simulink model "GMRforHapticsGuidance"  (R2012b)
settings: Solver=ode45  StartTime=0.0  StopTime=3  RelTol=1e-3
values from neighbouring files (symbols this model uses):
  sigmaGMR = [0.000145098551996 2.44735832162e-06 2.27908651022e-05 6.0139473564e-05 -2.08735404133e-05 -5.10583896034e-05 2.73525383282e-05 2.14077979945e-05 2.94117888322e-06 2.44735832162e-06 0.000208854387423 -0.000180360868853 ... (1134 elements, 9x9x14)]    [GMMData.mat]    (also in ModelTraining.m = reshape( covMatrices, [ numVar numVar 1 * numGauss ] ); ModelTraining2gestures.m = sigma; ModelTraining2gesturesZoom.m = sigma; ModelTraining2gesturesv1.m = sigma)
undefined symbols (not defined in the file or in its folder): B1, sigbuilder_block
settings Model: Creator=cperez  LastModifiedBy=andre
settings DataIOCC: SignalLoggingSaveFormat=ModelDataLogs
settings OptimizationCC: ExpressionDepthLimit=128
settings DebuggingCC: MultiTaskDSMMsg=warning  MultiTaskCondExecSysMsg=none  StateNameClashWarn=none  StrictBusMsg=None
settings RTWCC: IncludeERTFirstTime=on
settings CodeAppCC: CustomSymbolStrType=$N$R$M_T  InternalIdentifier=Shortened

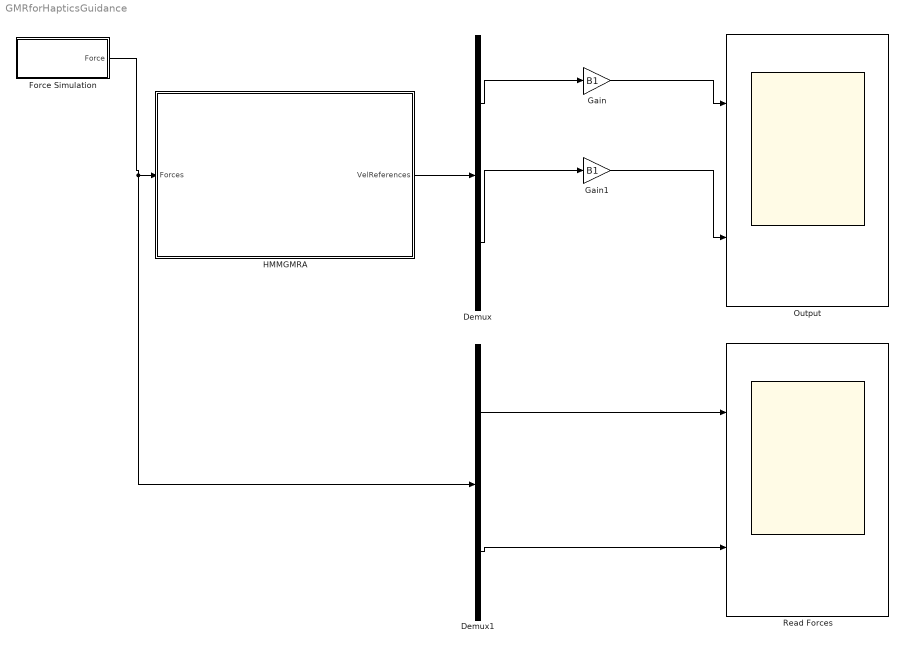
== system GMRforHapticsGuidance ==
  Demux : Demux  Outputs=2
  Demux1 : Demux  Outputs=2
  Force Simulation : Subsystem
  Gain : Gain  Gain=B1
  Gain1 : Gain  Gain=B1
  HMMGMRA : Subsystem
  Output : Scope  NumInputPorts=2
      settings: YMin=-5~-5  YMax=5~5
  Read Forces : Scope  NumInputPorts=2
      settings: YMin=-5~-5  YMax=5~5
  wires:
  HMMGMRA/1(VelReferences) -> Demux/1
  Demux/1 -> Gain/1
  Demux/2 -> Gain1/1
  Gain/1 -> Output/1
  Gain1/1 -> Output/2
  Demux1/1 -> Read Forces/1
  Demux1/2 -> Read Forces/2
  Force Simulation/1(Force) -> Demux1/1, HMMGMRA/1(Forces)

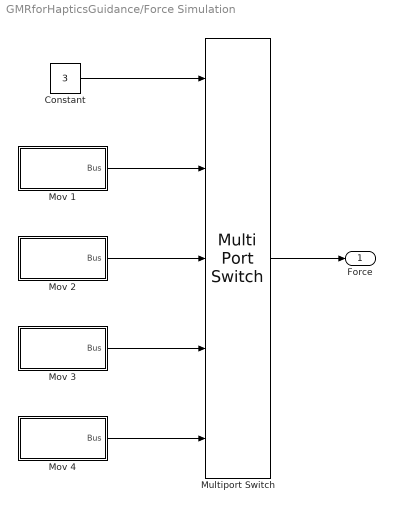
== system GMRforHapticsGuidance/Force Simulation ==
  Constant : Constant  Value=3
  Mov 1 : Subsystem  Tag=STV Subsys  LoadFcn=sigbuilder_block('load');  StartFcn=sigbuilder_block('start');  StopFcn=sigbuilder_block('stop');  ClipboardFcn=sigbuilder_block('clipboard');  mask(Sigbuilder block){}
      mask help: Simulink:masks:SigbuilderBlock_MD
      mask init:
      | if ~strcmp(get_param(bdroot(gcbh),'SimulationStatus'),'stopped') tuvar = sigbuilder_block('maskInit'); end
      settings: CopyFcn=sigbuilder_block('copy');  DeleteFcn=sigbuilder_block('delete');  ModelCloseFcn=sigbuilder_block('modelClose');  PreSaveFcn=sigbuilder_block('preSave');  PauseFcn=sigbuilder_block('pause');  ContinueFcn=sigbuilder_block('continue');  NameChangeFcn=sigbuilder_block('namechange');  OpenFcn=sigbuilder_block('open',[6 28.5 1428 718.5 ]);  CloseFcn=sigbuilder_block('close');
      mask Display: plot(0, 0, 100, 100,[2, 2, 32, 32, 2], [68, 8, 8, 68, 68],[32, 2], [38, 38], [32, 19, 2],[53, 60, 44], [32, 17, 17, 2],[16, 16, 31, 31]);txt = getActiveGroup(gcbh);text(2, 100, txt,'verticalAlignment', 'top');
  Mov 2 : Subsystem  Tag=STV Subsys  LoadFcn=sigbuilder_block('load');  StartFcn=sigbuilder_block('start');  StopFcn=sigbuilder_block('stop');  ClipboardFcn=sigbuilder_block('clipboard');  mask(Sigbuilder block){}
      mask help: Simulink:masks:SigbuilderBlock_MD
      mask init:
      | if ~strcmp(get_param(bdroot(gcbh),'SimulationStatus'),'stopped') tuvar = sigbuilder_block('maskInit'); end
      settings: CopyFcn=sigbuilder_block('copy');  DeleteFcn=sigbuilder_block('delete');  ModelCloseFcn=sigbuilder_block('modelClose');  PreSaveFcn=sigbuilder_block('preSave');  PauseFcn=sigbuilder_block('pause');  ContinueFcn=sigbuilder_block('continue');  NameChangeFcn=sigbuilder_block('namechange');  OpenFcn=sigbuilder_block('open',[6 28.5 1428 718.5 ]);  CloseFcn=sigbuilder_block('close');
      mask Display: plot(0, 0, 100, 100,[2, 2, 32, 32, 2], [68, 8, 8, 68, 68],[32, 2], [38, 38], [32, 19, 2],[53, 60, 44], [32, 17, 17, 2],[16, 16, 31, 31]);txt = getActiveGroup(gcbh);text(2, 100, txt,'verticalAlignment', 'top');
  Mov 3 : Subsystem  Tag=STV Subsys  LoadFcn=sigbuilder_block('load');  StartFcn=sigbuilder_block('start');  StopFcn=sigbuilder_block('stop');  ClipboardFcn=sigbuilder_block('clipboard');  mask(Sigbuilder block){}
      mask help: Simulink:masks:SigbuilderBlock_MD
      mask init:
      | if ~strcmp(get_param(bdroot(gcbh),'SimulationStatus'),'stopped') tuvar = sigbuilder_block('maskInit'); end
      settings: CopyFcn=sigbuilder_block('copy');  DeleteFcn=sigbuilder_block('delete');  ModelCloseFcn=sigbuilder_block('modelClose');  PreSaveFcn=sigbuilder_block('preSave');  PauseFcn=sigbuilder_block('pause');  ContinueFcn=sigbuilder_block('continue');  NameChangeFcn=sigbuilder_block('namechange');  OpenFcn=sigbuilder_block('open',[6 28.5 1428 718.5 ]);  CloseFcn=sigbuilder_block('close');
      mask Display: plot(0, 0, 100, 100,[2, 2, 32, 32, 2], [68, 8, 8, 68, 68],[32, 2], [38, 38], [32, 19, 2],[53, 60, 44], [32, 17, 17, 2],[16, 16, 31, 31]);txt = getActiveGroup(gcbh);text(2, 100, txt,'verticalAlignment', 'top');
  Mov 4 : Subsystem  Tag=STV Subsys  LoadFcn=sigbuilder_block('load');  StartFcn=sigbuilder_block('start');  StopFcn=sigbuilder_block('stop');  ClipboardFcn=sigbuilder_block('clipboard');  mask(Sigbuilder block){}
      mask help: Simulink:masks:SigbuilderBlock_MD
      mask init:
      | if ~strcmp(get_param(bdroot(gcbh),'SimulationStatus'),'stopped') tuvar = sigbuilder_block('maskInit'); end
      settings: CopyFcn=sigbuilder_block('copy');  DeleteFcn=sigbuilder_block('delete');  ModelCloseFcn=sigbuilder_block('modelClose');  PreSaveFcn=sigbuilder_block('preSave');  PauseFcn=sigbuilder_block('pause');  ContinueFcn=sigbuilder_block('continue');  NameChangeFcn=sigbuilder_block('namechange');  OpenFcn=sigbuilder_block('open',[6 28.5 1428 718.5 ]);  CloseFcn=sigbuilder_block('close');
      mask Display: plot(0, 0, 100, 100,[2, 2, 32, 32, 2], [68, 8, 8, 68, 68],[32, 2], [38, 38], [32, 19, 2],[53, 60, 44], [32, 17, 17, 2],[16, 16, 31, 31]);txt = getActiveGroup(gcbh);text(2, 100, txt,'verticalAlignment', 'top');
  Multiport Switch : MultiPortSwitch  Inputs=4
  Force : Outport
  wires:
  Multiport Switch/1 -> Force/1
  Constant/1 -> Multiport Switch/1
  Mov 1/1(Bus) -> Multiport Switch/2
  Mov 2/1(Bus) -> Multiport Switch/3
  Mov 3/1(Bus) -> Multiport Switch/4
  Mov 4/1(Bus) -> Multiport Switch/5

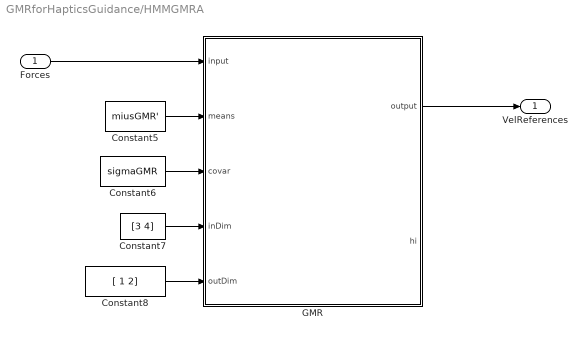
== system GMRforHapticsGuidance/HMMGMRA ==
  Forces : Inport
  Constant5 : Constant  Value=miusGMR'
  Constant6 : Constant  Value=sigmaGMR
  Constant7 : Constant  Value=[3 4]
  Constant8 : Constant  Value=[ 1 2]
  GMR : MATLAB Function  TreatAsAtomicUnit=on
  VelReferences : Outport
  wires:
  GMR/1(output) -> VelReferences/1
  Forces/1 -> GMR/1(input)
  Constant5/1 -> GMR/2(means)
  Constant6/1 -> GMR/3(covar)
  Constant7/1 -> GMR/4(inDim)
  Constant8/1 -> GMR/5(outDim)

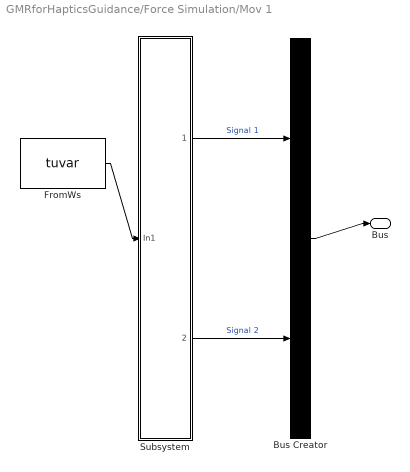
== system GMRforHapticsGuidance/Force Simulation/Mov 1 ==
  Bus Creator : BusCreator  Tag=Bus Creator  Inputs=2
  FromWs : FromWorkspace  Tag=STV FromWs  VariableName=tuvar  SampleTime=0
      SigBuilderData=|
      | common.afterFinalStr = 'Extrapolate'
      | common.sampleTime = 0
      | dataSet.timeRange = [0 3]
      | dataSet.name = 'Group 1'
      | sbobj.Groups.Name = 'Group 1'
      | sbobj.Groups.Signals(1).Name = 'Signal 1'
      | sbobj.Groups.Signals(1).XData = [0 3]
      | sbobj.Groups.Signals(1).YData = [2 0]
      | sbobj.Groups.Signals(2).Name = 'Signal 2'
      | sbobj.Groups.Signals(2).XData = [0 3]
      | sbobj.Groups.Signals(2).YData = [0 0]
      | sbobj.Groups.TimeRange = [0 3]
  Subsystem : Subsystem
  Bus : Outport
  wires:
  FromWs/1 -> Subsystem/1(In1)
  Subsystem/1(Signal 1) -> Bus Creator/1  "Signal 1"
  Subsystem/2(Signal 2) -> Bus Creator/2  "Signal 2"
  Bus Creator/1 -> Bus/1

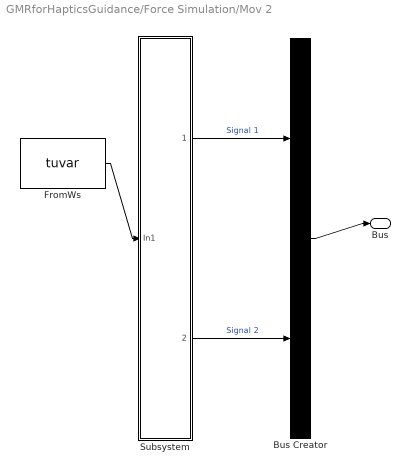
== system GMRforHapticsGuidance/Force Simulation/Mov 2 ==
  Bus Creator : BusCreator  Tag=Bus Creator  Inputs=2
  FromWs : FromWorkspace  Tag=STV FromWs  VariableName=tuvar  SampleTime=0
      SigBuilderData=|
      | common.afterFinalStr = 'Extrapolate'
      | common.sampleTime = 0
      | dataSet.timeRange = [0 3]
      | dataSet.name = 'Group 1'
      | sbobj.Groups.Name = 'Group 1'
      | sbobj.Groups.Signals(1).Name = 'Signal 1'
      | sbobj.Groups.Signals(1).XData = [0 3]
      | sbobj.Groups.Signals(1).YData = [-2 0]
      | sbobj.Groups.Signals(2).Name = 'Signal 2'
      | sbobj.Groups.Signals(2).XData = [0 3]
      | sbobj.Groups.Signals(2).YData = [0 0]
      | sbobj.Groups.TimeRange = [0 3]
  Subsystem : Subsystem
  Bus : Outport
  wires:
  FromWs/1 -> Subsystem/1(In1)
  Subsystem/1(Signal 1) -> Bus Creator/1  "Signal 1"
  Subsystem/2(Signal 2) -> Bus Creator/2  "Signal 2"
  Bus Creator/1 -> Bus/1

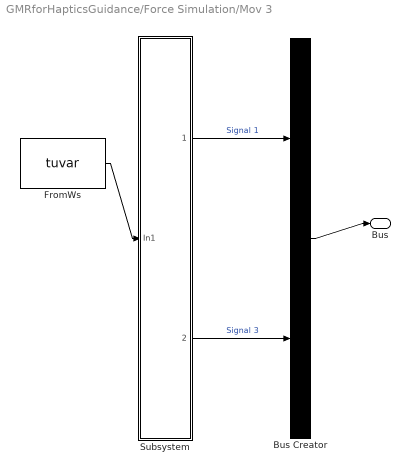
== system GMRforHapticsGuidance/Force Simulation/Mov 3 ==
  Bus Creator : BusCreator  Tag=Bus Creator  Inputs=2
  FromWs : FromWorkspace  Tag=STV FromWs  VariableName=tuvar  SampleTime=0
      SigBuilderData=|
      | common.afterFinalStr = 'Extrapolate'
      | common.sampleTime = 0
      | dataSet.timeRange = [0 3]
      | dataSet.name = 'Group 1'
      | sbobj.Groups.Name = 'Group 1'
      | sbobj.Groups.Signals(1).Name = 'Signal 1'
      | sbobj.Groups.Signals(1).XData = [0 3]
      | sbobj.Groups.Signals(1).YData = [0 0]
      | sbobj.Groups.Signals(2).Name = 'Signal 3'
      | sbobj.Groups.Signals(2).XData = [0 3]
      | sbobj.Groups.Signals(2).YData = [-2 0]
      | sbobj.Groups.TimeRange = [0 3]
  Subsystem : Subsystem
  Bus : Outport
  wires:
  FromWs/1 -> Subsystem/1(In1)
  Subsystem/1(Signal 1) -> Bus Creator/1  "Signal 1"
  Bus Creator/1 -> Bus/1
  Subsystem/2(Signal 3) -> Bus Creator/2  "Signal 3"

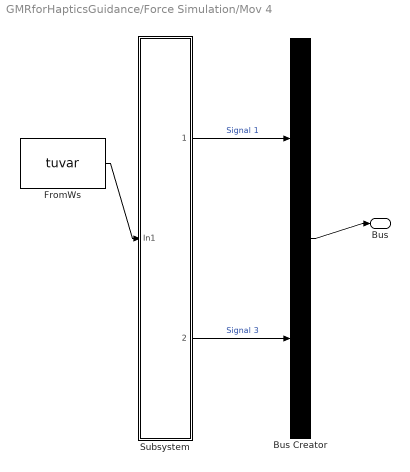
== system GMRforHapticsGuidance/Force Simulation/Mov 4 ==
  Bus Creator : BusCreator  Tag=Bus Creator  Inputs=2
  FromWs : FromWorkspace  Tag=STV FromWs  VariableName=tuvar  SampleTime=0
      SigBuilderData=|
      | common.afterFinalStr = 'Extrapolate'
      | common.sampleTime = 0
      | dataSet.timeRange = [0 3]
      | dataSet.name = 'Group 1'
      | sbobj.Groups.Name = 'Group 1'
      | sbobj.Groups.Signals(1).Name = 'Signal 1'
      | sbobj.Groups.Signals(1).XData = [0 3]
      | sbobj.Groups.Signals(1).YData = [0 0]
      | sbobj.Groups.Signals(2).Name = 'Signal 3'
      | sbobj.Groups.Signals(2).XData = [0 3]
      | sbobj.Groups.Signals(2).YData = [2 0]
      | sbobj.Groups.TimeRange = [0 3]
  Subsystem : Subsystem
  Bus : Outport
  wires:
  FromWs/1 -> Subsystem/1(In1)
  Subsystem/1(Signal 1) -> Bus Creator/1  "Signal 1"
  Bus Creator/1 -> Bus/1
  Subsystem/2(Signal 3) -> Bus Creator/2  "Signal 3"

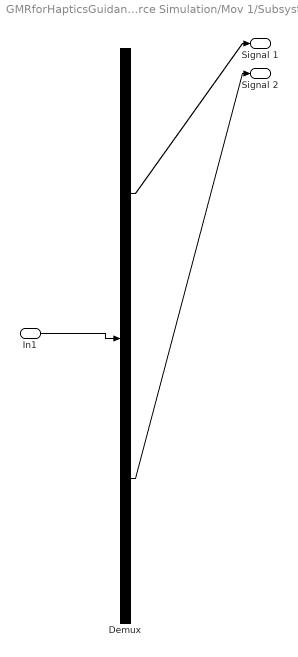
== system GMRforHapticsGuidance/Force Simulation/Mov 1/Subsystem ==
  In1 : Inport
  Demux : Demux  Tag=STV Demux  Outputs=2
  Signal 1 : Outport  Tag=STV Outport
  Signal 2 : Outport  Tag=STV Outport  Port=2
  wires:
  Demux/1 -> Signal 1/1
  Demux/2 -> Signal 2/1
  In1/1 -> Demux/1

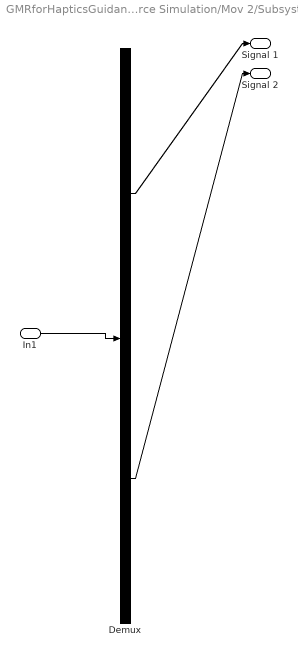
== system GMRforHapticsGuidance/Force Simulation/Mov 2/Subsystem ==
  In1 : Inport
  Demux : Demux  Tag=STV Demux  Outputs=2
  Signal 1 : Outport  Tag=STV Outport
  Signal 2 : Outport  Tag=STV Outport  Port=2
  wires:
  Demux/1 -> Signal 1/1
  Demux/2 -> Signal 2/1
  In1/1 -> Demux/1

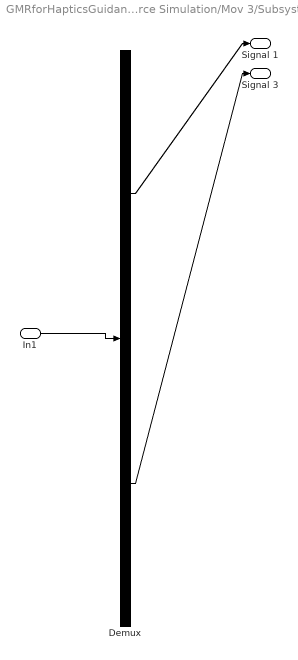
== system GMRforHapticsGuidance/Force Simulation/Mov 3/Subsystem ==
  In1 : Inport
  Demux : Demux  Tag=STV Demux  Outputs=2
  Signal 1 : Outport  Tag=STV Outport
  Signal 3 : Outport  Tag=STV Outport  Port=2
  wires:
  Demux/1 -> Signal 1/1
  In1/1 -> Demux/1
  Demux/2 -> Signal 3/1

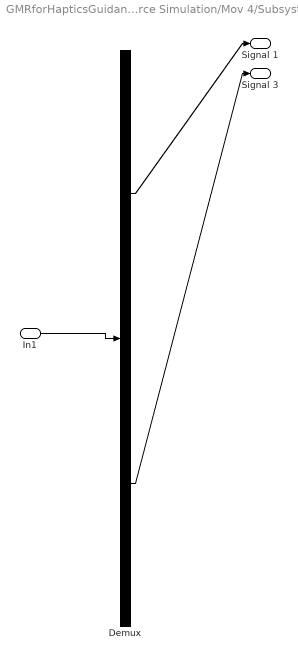
== system GMRforHapticsGuidance/Force Simulation/Mov 4/Subsystem ==
  In1 : Inport
  Demux : Demux  Tag=STV Demux  Outputs=2
  Signal 1 : Outport  Tag=STV Outport
  Signal 3 : Outport  Tag=STV Outport  Port=2
  wires:
  Demux/1 -> Signal 1/1
  In1/1 -> Demux/1
  Demux/2 -> Signal 3/1

== matlab function GMRforHapticsGuidance/HMMGMRA/GMR ==
  data: input input; output output; means input; covar input; inDim input; outDim input; hi output
function [ output, hi ] = gaussianMixtureRegression( input, means, ...
                              covar, inDim, outDim)

% This function carries out the Gaussian Mixture Regression from which it 
% is possible to obtain a serie of expected values for output (predictions)
% given a set of query points. The function develops the following steps:
%
% 1). Defines means and covariance matrices for P(x,y|j).
% 2). Computes the conditional expectation Å· and variance of y given x, for
%     each gaussian component.
% 3). Computes responsibilities of each gaussian component of producing
%     given x.
% 4). Computes the conditional expectation Å· and variance of y given x of
%     the entire mixture.
%
% The function gets as parameters:
% - input:  Query points (NxI)
% - means:  Means from GMM (KxZ)
% - covar:  Covariance matrices from GMM (ZxZxK)
% - inDim:  Vector indicating input dimensions (1xI)
% - outDim: Vector indicating output dimensions (1xO)
% 
% where
% - N: Number of query points
% - I: # Input variables
% - O: # Output variables
% - K: # Gaussian components
% - Z: I + O
                          
%% * * * Defining means and covariances with respect of inputs/outputs * * *
% When the probability P(x,y|j) is expressed as a normal pdf, it is 
% necessary to define:
% miu_j : [ miu_xj ; miu:yj ] 
% Cov_j : [ Cov_xxj Cov_xyj ; Cov_yxj Cov_yyj ] ;

% Means (miu)
miuInput    =   means( :, inDim ) ;
miuOutput   =   means( :, outDim ) ;

% Covariances (sigma)
covInput    =   covar( inDim, inDim, : ) ;
covOutput   =   covar( outDim, outDim, : ) ;
covInOut    =   covar( inDim, outDim, : ) ;
covOutIn    =   covar( outDim, inDim, : ) ;
                          

%% * * * Computing the conditional expectation and variance given input * * *                            
% numPts      =   size( input, 1 ) ;      % Number of query points
numGauss    =   size( means, 1 ) ;      % Number of gaussians
numOutputs  =   length( outDim ) ;     % Number of output dimensions

condY       =   zeros( numOutputs, numGauss ) ;

input=input';
% Conditional expectation Å·i for every query points 
for i = 1 : numGauss
    % Computing difference between each input point and input mean (miu_xj)
    diff        =   ( input - ones( 1, 1 ) * miuInput( i, : ) )' ;
    % Computing conditional expectation Å· for j-th gaussian
    condY(:,i)=   ( ones( 1, 1 ) * miuOutput( i, : ) ) + ...
                    ( ( covOutIn( :, :, i ) / covInput( :, :, i ) ) * diff )';
end

condSigma   =   zeros( numOutputs, numOutputs, numGauss ) ;
% Conditional covariance sigma_j (estimated)
for i = 1 : numGauss
    condSigma( :, :, i )    =   covOutput( :, :, i ) - ...
        ( covOutIn( :, :, i ) / covInput( :, :, i ) ) * covInOut( :, :, i ) ;
end


%% * * * * Computing responsibilities of each Gaussian given input * * * *
% Conditional probability of x given j-th gaussian
pxi     =   zeros( numGauss, 1 ) ;
for i = 1 : numGauss
    pxi( i, : ) =   gaussianPDF( input, miuInput( i, : ), covInput( :, :, i ) ) ;
end

% Responsibilities for each gaussian
hi  =   zeros( numGauss, 1 ) ;
for i = 1 : 1
    hi( :, i )  =   pxi( :, i ) ./ sum( pxi( :, i ) ) ;
end


%% * * * Computing conditional expectation and variance of the mixture * * *
% Conditional expectation Å· of the resulting mixture given input
condYmixt   =   zeros( numOutputs, numGauss ) ;
for i = 1 : numGauss
    condYmixt( :, i )    =   condYmixt( :, i ) + ...
        ( ( hi( i, : )' .* condY( :, i ) ) ) ;
end
output  =   sum( condYmixt, 2 ) ;
